simulink model "dados_simulados"  (R2020b)
settings: Solver=VariableStepAuto  StartTime=0.0  StopTime=30  RelTol=1e-3
values from neighbouring files (symbols this model uses):
  C = [1 0 0 ;0 1 0 ]    [experinces.m]    (also in main.m = [1 0])
  Q = diag([0 0.005 1*10^-4 ])    [experinces.m]    (also in main.m = 0.005*[0 0; 0 1])
  R = diag([0.0005/150 0.05/150])    [experinces.m]    (also in main.m = 3.33333333333e-05)
settings Model: Creator=renato  LastModifiedBy=renato

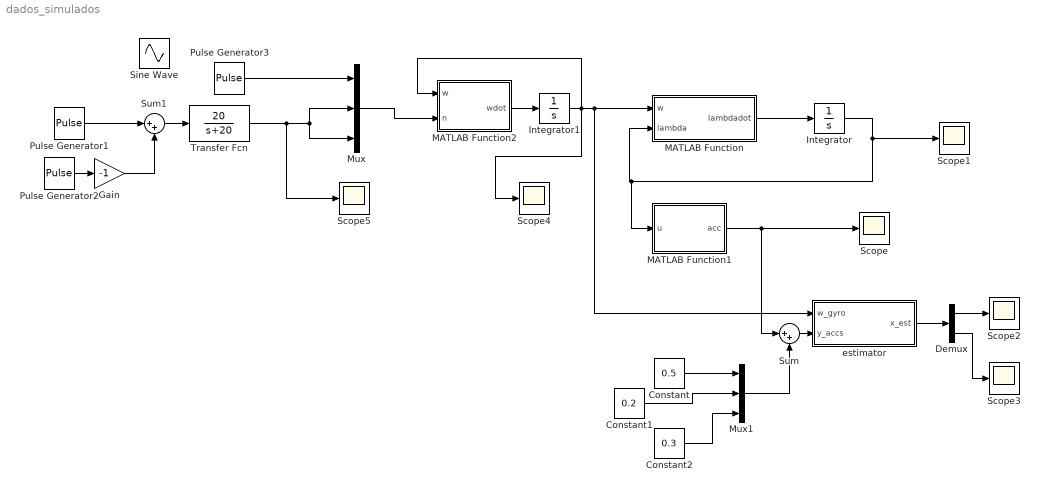
== system dados_simulados ==
  Constant : Constant  Value=0.5
  Constant1 : Constant  Value=0.2
  Constant2 : Constant  Value=0.3
  Demux : Demux  Outputs=[3 3]
  Gain : Gain  Gain=-1
  Integrator : Integrator  InitialCondition=[0;0;0]
  Integrator1 : Integrator  InitialCondition=[0;0;0]
  MATLAB Function : MATLAB Function  TreatAsAtomicUnit=on
  MATLAB Function1 : MATLAB Function  TreatAsAtomicUnit=on
  MATLAB Function2 : MATLAB Function  TreatAsAtomicUnit=on
  Mux : Mux  Inputs=3
  Mux1 : Mux  Inputs=3
  Pulse Generator1 : DiscretePulseGenerator  PulseType=Time based  Amplitude=0.001  Period=30  PulseWidth=10  PhaseDelay=5
  Pulse Generator2 : DiscretePulseGenerator  PulseType=Time based  Amplitude=0.01  Period=30  PulseWidth=10  PhaseDelay=20
  Pulse Generator3 : DiscretePulseGenerator  PulseType=Time based  Amplitude=0.001  Period=30  PulseWidth=10  PhaseDelay=5
  Scope{,1..5} (6 alike) : Scope
  Sine Wave : Sin  Amplitude=0.1  SampleTime=0
  Sum : Sum  Inputs=|++
  Sum1 : Sum  Inputs=|++
  Transfer Fcn : TransferFcn  Numerator=[20]  Denominator=[1 20]
  estimator : Subsystem
  wires:
  MATLAB Function/1(lambdadot) -> Integrator/1
  Integrator/1 -> Scope1/1, MATLAB Function1/1(u), MATLAB Function/2(lambda)
  MATLAB Function1/1(acc) -> Sum/1, Scope/1
  estimator/1(x_est) -> Demux/1
  Demux/1 -> Scope2/1
  Demux/2 -> Scope3/1
  Sum/1 -> estimator/2(y_accs)
  Mux1/1 -> Sum/2
  Constant/1 -> Mux1/1
  Constant1/1 -> Mux1/2
  Constant2/1 -> Mux1/3
  Integrator1/1 -> Scope4/1, MATLAB Function2/1(w), estimator/1(w_gyro), MATLAB Function/1(w)
  Mux/1 -> MATLAB Function2/2(n)
  MATLAB Function2/1(wdot) -> Integrator1/1
  Transfer Fcn/1 -> Scope5/1, Mux/3, Mux/2
  Pulse Generator2/1 -> Gain/1
  Gain/1 -> Sum1/2
  Pulse Generator1/1 -> Sum1/1
  Sum1/1 -> Transfer Fcn/1
  Pulse Generator3/1 -> Mux/1

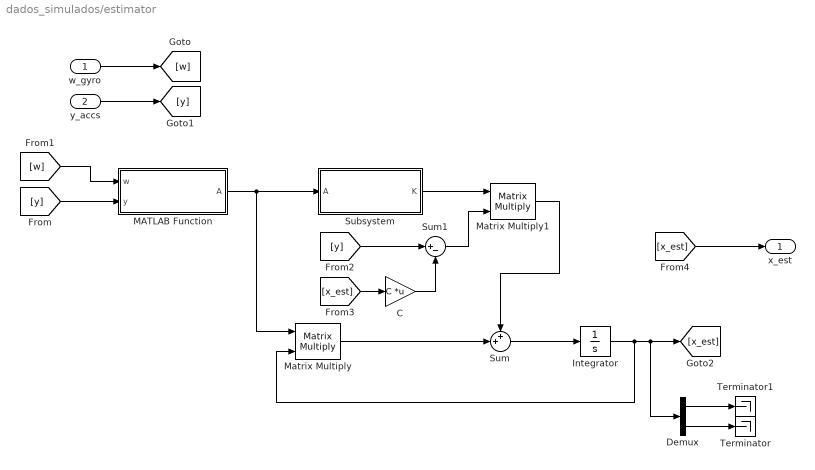
== system dados_simulados/estimator ==
  w_gyro : Inport
  y_accs : Inport  Port=2
  C : Gain  Gain=C  Multiplication=Matrix(K*u)
  Demux : Demux  Outputs=[3 3]
  Integrator : Integrator
  MATLAB Function : MATLAB Function  TreatAsAtomicUnit=on
  Matrix Multiply : Product  Multiplication=Matrix(*)
  Matrix Multiply1 : Product  Multiplication=Matrix(*)
  Subsystem : Subsystem
  Sum : Sum  Inputs=++|
  Sum1 : Sum  Inputs=|+-
  Terminator : Terminator
  Terminator1 : Terminator
  x_est : Outport
  wires:
  Integrator/1 -> Demux/1, [x_est], Matrix Multiply/2
  Subsystem/1(K) -> Matrix Multiply1/1
  [x_est] -> C/1
  C/1 -> Sum1/2
  Sum/1 -> Integrator/1
  [y] -> MATLAB Function/2(y)
  [w] -> MATLAB Function/1(w)
  [y] -> Sum1/1
  Matrix Multiply1/1 -> Sum/1
  Sum1/1 -> Matrix Multiply1/2
  Matrix Multiply/1 -> Sum/2
  MATLAB Function/1(A) -> Subsystem/1(A), Matrix Multiply/1
  [x_est] -> x_est/1
  w_gyro/1 -> [w]
  y_accs/1 -> [y]
  Demux/2 -> Terminator/1
  Demux/1 -> Terminator1/1

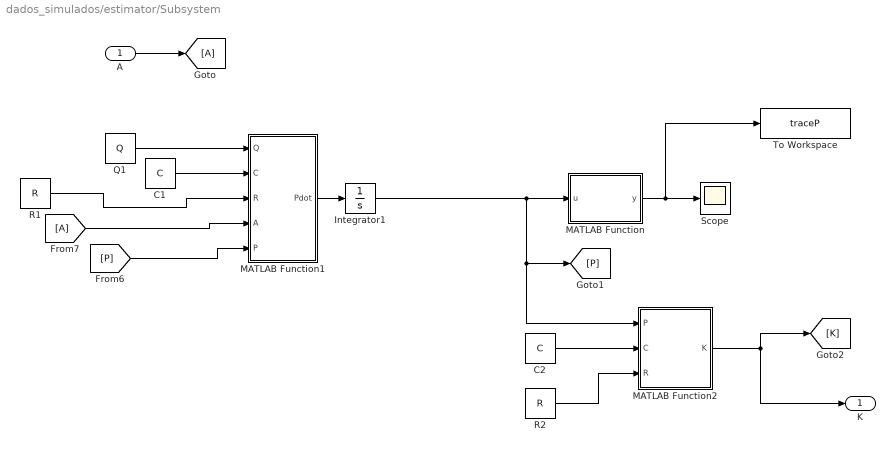
== system dados_simulados/estimator/Subsystem ==
  A : Inport
  C1 : Constant  Value=C
  C2 : Constant  Value=C
  Integrator1 : Integrator  InitialCondition=eye(6)
  MATLAB Function : MATLAB Function  TreatAsAtomicUnit=on
  MATLAB Function1 : MATLAB Function  TreatAsAtomicUnit=on
  MATLAB Function2 : MATLAB Function  TreatAsAtomicUnit=on
  Q1 : Constant  Value=Q
  R1 : Constant  Value=R
  R2 : Constant  Value=R
  Scope : Scope
  To Workspace : ToWorkspace  VariableName=traceP  SaveFormat=Timeseries  SampleTime=-1
  K : Outport
  wires:
  A/1 -> [A]
  MATLAB Function/1(y) -> To Workspace/1, Scope/1
  Q1/1 -> MATLAB Function1/1(Q)
  [P] -> MATLAB Function1/5(P)
  [A] -> MATLAB Function1/4(A)
  R1/1 -> MATLAB Function1/3(R)
  C1/1 -> MATLAB Function1/2(C)
  MATLAB Function1/1(Pdot) -> Integrator1/1
  Integrator1/1 -> MATLAB Function2/1(P), [P], MATLAB Function/1(u)
  C2/1 -> MATLAB Function2/2(C)
  R2/1 -> MATLAB Function2/3(R)
  MATLAB Function2/1(K) -> [K], K/1

== matlab function dados_simulados/MATLAB Function1 ==
  data: u input; acc output
function acc = fcn(u)
g=9.8;
x=-g*sin(u(1));
y=-g*cos(u(1))*sin(u(2));
z=-g*cos(u(1))*cos(u(2));
acc=[x;y;z];

== matlab function dados_simulados/MATLAB Function ==
  data: w input; lambdadot output; lambda input
function lambdadot = fcn(w,lambda)
Q=[1 ,sin(lambda(2))*tan(lambda(1)), cos(lambda(2))*tan(lambda(1));
    0, cos(lambda(2)), -sin(lambda(2));
    0, sin(lambda(2))/cos(lambda(1)), cos(lambda(2))/cos(lambda(1))];
%Q=eye(3)
lambdadot=Q*w;

== matlab function dados_simulados/estimator/MATLAB Function ==
  data: w input; A output; y input
function A = calculate_A(w, y)
    aux1 = -[0, -w(3), w(2); 
             w(3), 0, -w(1);
             -w(2), w(1), 0];
    aux2 = -[0, -y(3), y(2);
            y(3), 0, -y(1);
            -y(2), y(1), 0];   
    
A = [aux1 , aux2; zeros(3), zeros(3)];

== matlab function dados_simulados/estimator/Subsystem/MATLAB Function ==
  data: u input; y output
function y = fcn(u)

y = trace(u);

== matlab function dados_simulados/estimator/Subsystem/MATLAB Function1 ==
  data: Q input; Pdot output; C input; R input; A input; P input
function Pdot = fcn(Q,C,R,A,P)
    Pdot=A*P + P*A' +Q -P*C'/R*C*P;
end

== matlab function dados_simulados/estimator/Subsystem/MATLAB Function2 ==
  data: P input; K output; C input; R input
function K = fcn(P,C,R)
    K=P*C'/R;
end

== matlab function dados_simulados/MATLAB Function2 ==
  data: w input; wdot output; n input
function wdot = fcn(w, n)
aux=-[0, -w(3), w(2); w(3),0, -w(1);-w(2), w(1),0];
wdot=aux*w + n;
